simulink model "Q2b"  (R2022a)
settings: Solver=VariableStepAuto  StartTime=0.0  StopTime=12.0  RelTol=1e-3
settings Model: SnapshotInterval=1  Creator=Asus  LastModifiedBy=Asus

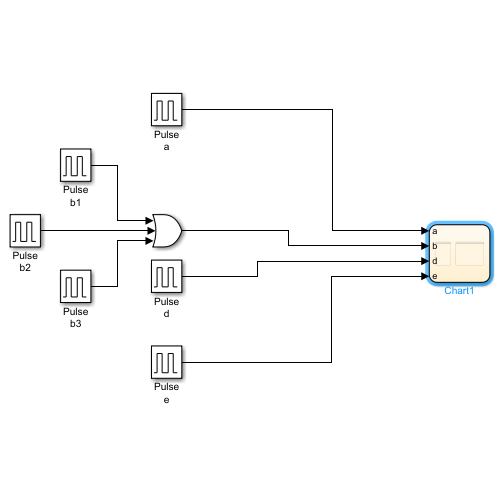
[thumbnail: Simulink's stored preview of the top-level diagram]
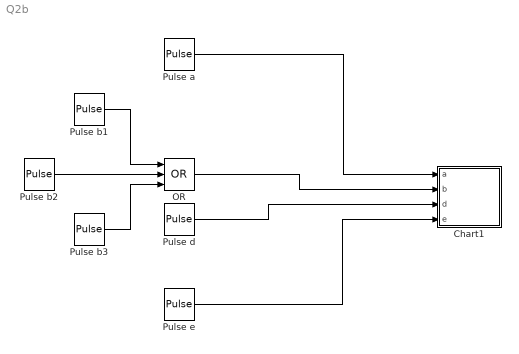
== system Q2b ==
  Chart1 : Stateflow chart  TreatAsAtomicUnit=on
  OR : Logic  Operator=OR  Inputs=3  IconShape=distinctive  AllPortsSameDT=off  OutDataTypeStr=boolean
  Pulse a : DiscretePulseGenerator  PulseType=Time based  Period=12  PhaseDelay=2
  Pulse b1 : DiscretePulseGenerator  PulseType=Time based  Period=12  PhaseDelay=12
  Pulse b2 : DiscretePulseGenerator  PulseType=Time based  Period=12  PhaseDelay=8
  Pulse b3 : DiscretePulseGenerator  PulseType=Time based  Period=12  PhaseDelay=4
  Pulse d : DiscretePulseGenerator  PulseType=Time based  Period=12  PhaseDelay=10
  Pulse e : DiscretePulseGenerator  PulseType=Time based  Period=12  PhaseDelay=6
  wires:
  Pulse b1/1 -> OR/1
  Pulse b2/1 -> OR/2
  Pulse e/1 -> Chart1/4(e)
  Pulse a/1 -> Chart1/1(a)
  Pulse b3/1 -> OR/3
  OR/1 -> Chart1/2(b)
  Pulse d/1 -> Chart1/3(d)

== stateflow chart Q2b/Chart1 ==
  state B [parallel]
    settings: executionOrder=2
    state one
    state two
    (default) -> one
    one -> two : [c]
    two -> one : [b && in(C.D.D2)]
  state C [parallel]
    settings: executionOrder=1
    state D
      state D1
      state D2
      (default) -> D1
      D1 -> D2 : [e]{c = 0}
      D2 -> D2 : [e]
    state G
    G -> D : [a]{c = 1}
    (default) -> G
    D -> G : [d]
  data: c local =0; a input; b input; d input; e input
